simulink model "guidanceNonLinearFede"  (R2020a)
settings: Solver=VariableStepAuto  StartTime=0.0  StopTime=10.0  RelTol=1e-3
values from neighbouring files (symbols this model uses):
  Ag = 1    [guidanceFede.m]
  alpha = 1    [guidanceFede.m]
  g = 9.8    [guidanceFede.m]
  ig1_init = 0    [guidanceFede.m]
  ig2_init = 0    [guidanceFede.m]
  ig3_init = 0    [guidanceFede.m]
  ig4_init = 0    [guidanceFede.m]
  ig5_init = 0    [guidanceFede.m]
  ig6_init = 0    [guidanceFede.m]
  Ipsi = 1    [guidanceFede.m]
  K = lqr(A,B,Q,R)    [guidanceFede.m]
  m = 1    [guidanceFede.m]
  mu0 = 1    [guidanceFede.m]
  Ng = 1    [guidanceFede.m]
  P1 = 1    [guidanceFede.m]
  P2 = 1    [guidanceFede.m]
  P3 = 1    [guidanceFede.m]
  P4 = 1    [guidanceFede.m]
  P5 = 1    [guidanceFede.m]
  P6 = 1    [guidanceFede.m]
  phi = 1    [guidanceFede.m]
  psi_init = 0.01*rand(1)    [guidanceFede.m]
  Ra = 1    [guidanceFede.m]
  vy_init = rand(1)    [guidanceFede.m]
  wpsi_init = 0.01*rand(1)    [guidanceFede.m]
  wtheta = 1    [guidanceFede.m]
  xB = 1    [guidanceFede.m]
  xe = [ ye; vye; psie; wpsie; ig1e; ig2e; ig3e; ig4e; ig5e; ig6e]    [guidanceFede.m]
  y_init = rand(1)    [guidanceFede.m]
  yB = 1    [guidanceFede.m]
settings Model: Creator=Federico  LastModifiedBy=Federico

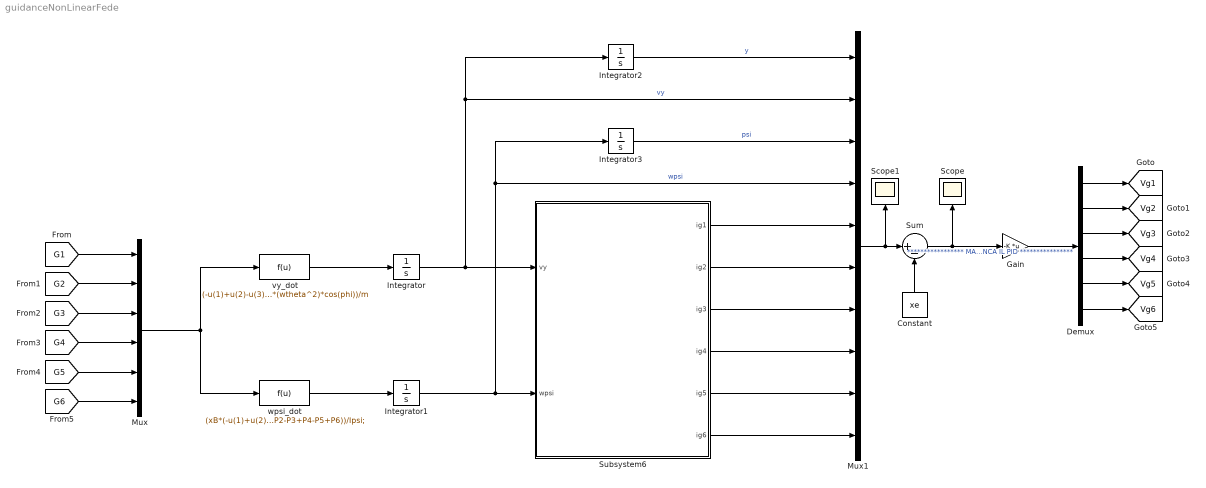
== system guidanceNonLinearFede ==
  Constant : Constant  Value=xe
  Demux : Demux  Outputs=6
  Gain : Gain  Gain=-K  Multiplication=Matrix(K*u)
  Integrator : Integrator  InitialCondition=vy_init
  Integrator1 : Integrator  InitialCondition=wpsi_init
  Integrator2 : Integrator  InitialCondition=y_init
  Integrator3 : Integrator  InitialCondition=psi_init
  Mux : Mux  Inputs=6
  Mux1 : Mux  Inputs=10
  Scope : Scope
  Scope1 : Scope
  Subsystem6 : Subsystem
  Sum : Sum  Inputs=|+-
  vy_dot : Fcn  Expr=(-u(1)+u(2)-u(3)+u(4)-u(5)+u(6)+m*g*sin(phi)-m*Ra*(wtheta^2)*cos(phi))/m
  wpsi_dot : Fcn  Expr=(xB*(-u(1)+u(2)+u(5)-u(6))+yB*(-P1+P2-P3+P4-P5+P6))/Ipsi;
  tag scope: Vg1=global, Vg2=global, Vg3=global, Vg4=global, Vg5=global, Vg6=global
  wires:
  vy_dot/1 -> Integrator/1
  wpsi_dot/1 -> Integrator1/1
  Integrator/1 -> Integrator2/1, Mux1/2, Subsystem6/1(vy)  "vy"
  Integrator1/1 -> Integrator3/1, Mux1/4, Subsystem6/2(wpsi)  "wpsi"
  Mux/1 -> wpsi_dot/1, vy_dot/1
  [G1] -> Mux/1
  [G2] -> Mux/2
  [G3] -> Mux/3
  [G4] -> Mux/4
  [G5] -> Mux/5
  [G6] -> Mux/6
  Integrator2/1 -> Mux1/1  "y"
  Integrator3/1 -> Mux1/3  "psi"
  Subsystem6/1(ig1) -> Mux1/5
  Subsystem6/2(ig2) -> Mux1/6
  Subsystem6/3(ig3) -> Mux1/7
  Subsystem6/4(ig4) -> Mux1/8
  Subsystem6/5(ig5) -> Mux1/9
  Subsystem6/6(ig6) -> Mux1/10
  Gain/1 -> Demux/1
  Demux/1 -> [Vg1]
  Demux/2 -> [Vg2]
  Demux/4 -> [Vg4]
  Demux/3 -> [Vg3]
  Demux/5 -> [Vg5]
  Demux/6 -> [Vg6]
  Mux1/1 -> Scope1/1, Sum/1
  Sum/1 -> Scope/1, Gain/1  "***************** MANCA IL PID ****************"
  Constant/1 -> Sum/2

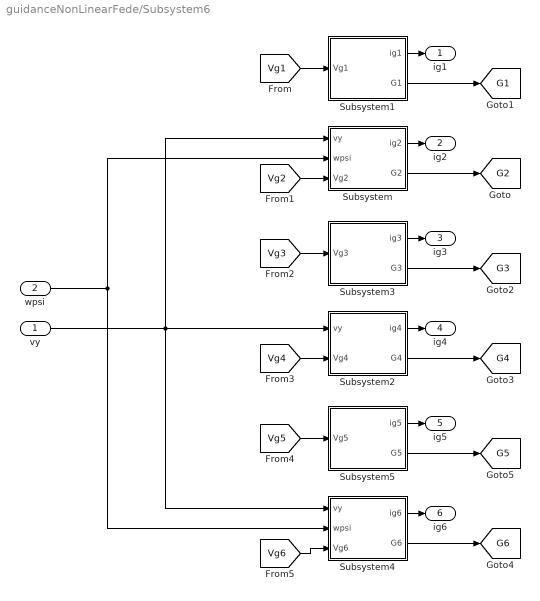
== system guidanceNonLinearFede/Subsystem6 ==
  vy : Inport
  wpsi : Inport  Port=2
  Subsystem : Subsystem
  Subsystem1 : Subsystem
  Subsystem2 : Subsystem
  Subsystem3 : Subsystem
  Subsystem4 : Subsystem
  Subsystem5 : Subsystem
  ig1 : Outport
  ig2 : Outport  Port=2
  ig3 : Outport  Port=3
  ig4 : Outport  Port=4
  ig5 : Outport  Port=5
  ig6 : Outport  Port=6
  tag scope: G1=global, G2=global, G3=global, G4=global, G5=global, G6=global
  wires:
  [Vg2] -> Subsystem/3(Vg2)
  [Vg3] -> Subsystem3/1(Vg3)
  Subsystem/2(G2) -> [G2]
  Subsystem3/2(G3) -> [G3]
  Subsystem2/2(G4) -> [G4]
  Subsystem/1(ig2) -> ig2/1
  Subsystem5/2(G5) -> [G5]
  Subsystem4/2(G6) -> [G6]
  Subsystem1/2(G1) -> [G1]
  Subsystem4/1(ig6) -> ig6/1
  vy/1 -> Subsystem/1(vy), Subsystem4/1(vy), Subsystem2/1(vy)
  Subsystem5/1(ig5) -> ig5/1
  Subsystem3/1(ig3) -> ig3/1
  wpsi/1 -> Subsystem4/2(wpsi), Subsystem/2(wpsi)
  Subsystem1/1(ig1) -> ig1/1
  Subsystem2/1(ig4) -> ig4/1
  [Vg6] -> Subsystem4/3(Vg6)
  [Vg1] -> Subsystem1/1(Vg1)
  [Vg4] -> Subsystem2/2(Vg4)
  [Vg5] -> Subsystem5/1(Vg5)

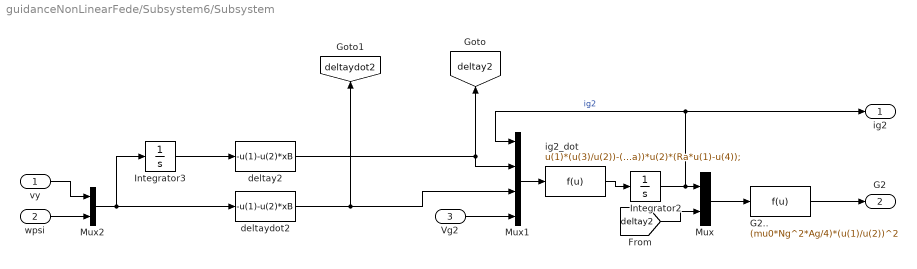
== system guidanceNonLinearFede/Subsystem6/Subsystem ==
  vy : Inport
  wpsi : Inport  Port=2
  Vg2 : Inport  Port=3
  G2.. : Fcn  Expr=(mu0*Ng^2*Ag/4)*(u(1)/u(2))^2
  Integrator2 : Integrator  InitialCondition=ig2_init
  Integrator3 : Integrator  InitialCondition=[vy_init; wpsi_init]
  Mux : Mux  Inputs=2
  Mux1 : Mux
  Mux2 : Mux  Inputs=2
  deltay2 : Fcn  Expr=-u(1)-u(2)*xB
  deltaydot2 : Fcn  Expr=-u(1)-u(2)*xB
  ig2_dot : Fcn  Expr=u(1)*(u(3)/u(2))-(2/(mu0*Ng*alpha))*u(2)*(Ra*u(1)-u(4));
  ig2 : Outport
  G2 : Outport  Port=2
  tag scope: deltay2=global, deltaydot2=global
  wires:
  ig2_dot/1 -> Integrator2/1
  G2../1 -> G2/1
  deltaydot2/1 -> Mux1/3, [deltaydot2]
  vy/1 -> Mux2/1
  Mux2/1 -> Integrator3/1, deltaydot2/1
  Vg2/1 -> Mux1/4
  Mux/1 -> G2../1
  Integrator2/1 -> ig2/1, Mux1/1, Mux/1  "ig2"
  wpsi/1 -> Mux2/2
  [deltay2] -> Mux/2
  Mux1/1 -> ig2_dot/1
  Integrator3/1 -> deltay2/1
  deltay2/1 -> [deltay2], Mux1/2

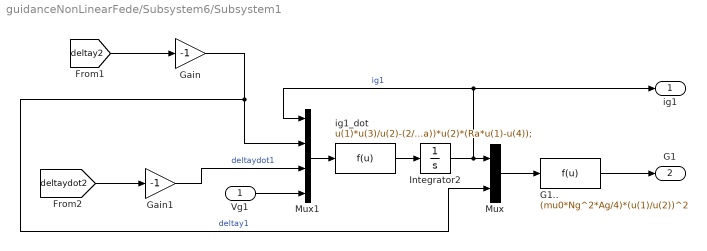
== system guidanceNonLinearFede/Subsystem6/Subsystem1 ==
  Vg1 : Inport
  G1.. : Fcn  Expr=(mu0*Ng^2*Ag/4)*(u(1)/u(2))^2
  Gain : Gain  Gain=-1
  Gain1 : Gain  Gain=-1
  Integrator2 : Integrator  InitialCondition=ig1_init
  Mux : Mux  Inputs=2
  Mux1 : Mux
  ig1_dot : Fcn  Expr=u(1)*u(3)/u(2)-(2/(mu0*Ng*alpha))*u(2)*(Ra*u(1)-u(4));
  ig1 : Outport
  G1 : Outport  Port=2
  wires:
  Mux1/1 -> ig1_dot/1
  Integrator2/1 -> Mux/1, Mux1/1, ig1/1  "ig1"
  Mux/1 -> G1../1
  Vg1/1 -> Mux1/4
  G1../1 -> G1/1
  ig1_dot/1 -> Integrator2/1
  [deltay2] -> Gain/1
  [deltaydot2] -> Gain1/1
  Gain/1 -> Mux1/2, Mux/2  "deltay1"
  Gain1/1 -> Mux1/3  "deltaydot1"

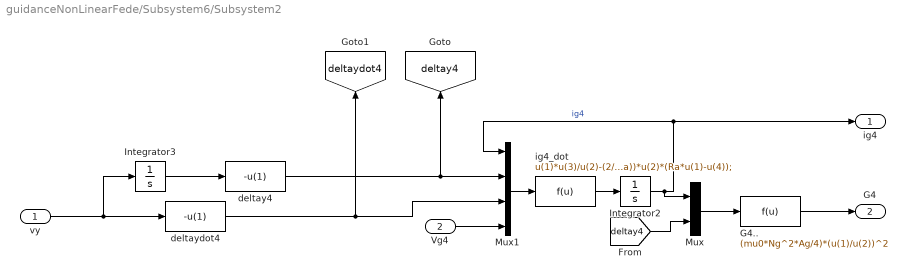
== system guidanceNonLinearFede/Subsystem6/Subsystem2 ==
  vy : Inport
  Vg4 : Inport  Port=2
  G4.. : Fcn  Expr=(mu0*Ng^2*Ag/4)*(u(1)/u(2))^2
  Integrator2 : Integrator  InitialCondition=ig4_init
  Integrator3 : Integrator  InitialCondition=vy_init
  Mux : Mux  Inputs=2
  Mux1 : Mux
  deltay4 : Fcn  Expr=-u(1)
  deltaydot4 : Fcn  Expr=-u(1)
  ig4_dot : Fcn  Expr=u(1)*u(3)/u(2)-(2/(mu0*Ng*alpha))*u(2)*(Ra*u(1)-u(4));
  ig4 : Outport
  G4 : Outport  Port=2
  tag scope: deltay4=global, deltaydot4=global
  wires:
  deltay4/1 -> [deltay4], Mux1/2
  Integrator3/1 -> deltay4/1
  Mux1/1 -> ig4_dot/1
  [deltay4] -> Mux/2
  Integrator2/1 -> Mux/1, Mux1/1, ig4/1  "ig4"
  Mux/1 -> G4../1
  Vg4/1 -> Mux1/4
  deltaydot4/1 -> Mux1/3, [deltaydot4]
  G4../1 -> G4/1
  ig4_dot/1 -> Integrator2/1
  vy/1 -> Integrator3/1, deltaydot4/1

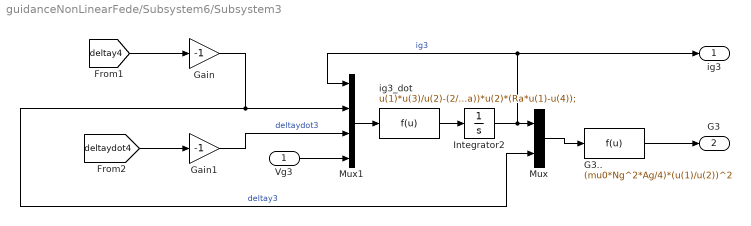
== system guidanceNonLinearFede/Subsystem6/Subsystem3 ==
  Vg3 : Inport
  G3.. : Fcn  Expr=(mu0*Ng^2*Ag/4)*(u(1)/u(2))^2
  Gain : Gain  Gain=-1
  Gain1 : Gain  Gain=-1
  Integrator2 : Integrator  InitialCondition=ig3_init
  Mux : Mux  Inputs=2
  Mux1 : Mux
  ig3_dot : Fcn  Expr=u(1)*u(3)/u(2)-(2/(mu0*Ng*alpha))*u(2)*(Ra*u(1)-u(4));
  ig3 : Outport
  G3 : Outport  Port=2
  wires:
  Gain1/1 -> Mux1/3  "deltaydot3"
  Gain/1 -> Mux1/2, Mux/2  "deltay3"
  [deltaydot4] -> Gain1/1
  [deltay4] -> Gain/1
  ig3_dot/1 -> Integrator2/1
  G3../1 -> G3/1
  Vg3/1 -> Mux1/4
  Mux/1 -> G3../1
  Integrator2/1 -> ig3/1, Mux1/1, Mux/1  "ig3"
  Mux1/1 -> ig3_dot/1

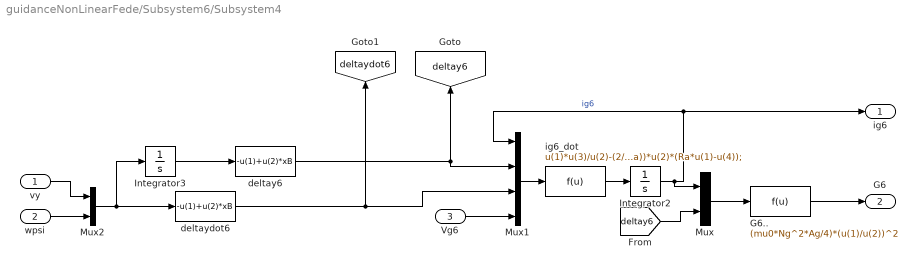
== system guidanceNonLinearFede/Subsystem6/Subsystem4 ==
  vy : Inport
  wpsi : Inport  Port=2
  Vg6 : Inport  Port=3
  G6.. : Fcn  Expr=(mu0*Ng^2*Ag/4)*(u(1)/u(2))^2
  Integrator2 : Integrator  InitialCondition=ig6_init
  Integrator3 : Integrator  InitialCondition=[vy_init; wpsi_init]
  Mux : Mux  Inputs=2
  Mux1 : Mux
  Mux2 : Mux  Inputs=2
  deltay6 : Fcn  Expr=-u(1)+u(2)*xB
  deltaydot6 : Fcn  Expr=-u(1)+u(2)*xB
  ig6_dot : Fcn  Expr=u(1)*u(3)/u(2)-(2/(mu0*Ng*alpha))*u(2)*(Ra*u(1)-u(4));
  ig6 : Outport
  G6 : Outport  Port=2
  tag scope: deltay6=global, deltaydot6=global
  wires:
  ig6_dot/1 -> Integrator2/1
  G6../1 -> G6/1
  deltaydot6/1 -> Mux1/3, [deltaydot6]
  vy/1 -> Mux2/1
  Mux2/1 -> Integrator3/1, deltaydot6/1
  Vg6/1 -> Mux1/4
  Mux/1 -> G6../1
  Integrator2/1 -> ig6/1, Mux1/1, Mux/1  "ig6"
  wpsi/1 -> Mux2/2
  [deltay6] -> Mux/2
  Mux1/1 -> ig6_dot/1
  Integrator3/1 -> deltay6/1
  deltay6/1 -> Mux1/2, [deltay6]

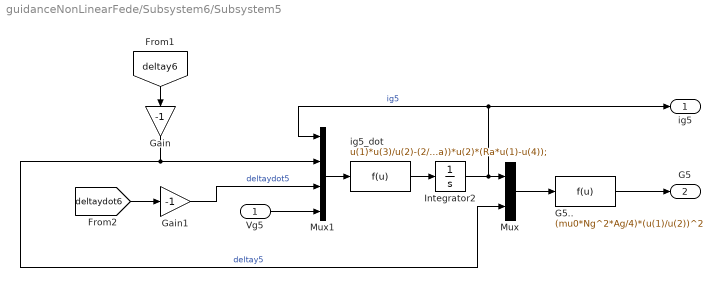
== system guidanceNonLinearFede/Subsystem6/Subsystem5 ==
  Vg5 : Inport
  G5.. : Fcn  Expr=(mu0*Ng^2*Ag/4)*(u(1)/u(2))^2
  Gain : Gain  Gain=-1
  Gain1 : Gain  Gain=-1
  Integrator2 : Integrator  InitialCondition=ig5_init
  Mux : Mux  Inputs=2
  Mux1 : Mux
  ig5_dot : Fcn  Expr=u(1)*u(3)/u(2)-(2/(mu0*Ng*alpha))*u(2)*(Ra*u(1)-u(4));
  ig5 : Outport
  G5 : Outport  Port=2
  wires:
  Mux1/1 -> ig5_dot/1
  Integrator2/1 -> Mux/1, Mux1/1, ig5/1  "ig5"
  Mux/1 -> G5../1
  Vg5/1 -> Mux1/4
  G5../1 -> G5/1
  ig5_dot/1 -> Integrator2/1
  [deltay6] -> Gain/1
  [deltaydot6] -> Gain1/1
  Gain/1 -> Mux/2, Mux1/2  "deltay5"
  Gain1/1 -> Mux1/3  "deltaydot5"
